simulink model "No"  (R2018b)
settings: Solver=VariableStepAuto  StartTime=0.0  StopTime=10.0  RelTol=1e-3
settings Model: Creator=kekos  LastModifiedBy=kekos

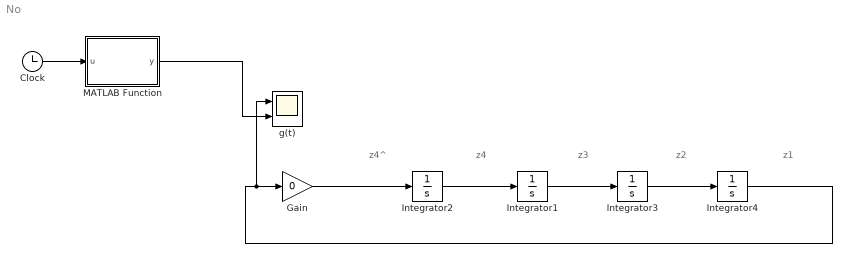
== system No ==
  note: z1
  note: z2
  note: z3
  note: z4
  note: z4^
  Clock : Clock
  Gain : Gain  Gain=0
  Integrator1 : Integrator
  Integrator2 : Integrator  InitialCondition=18
  Integrator3 : Integrator  InitialCondition=2
  Integrator4 : Integrator  InitialCondition=1
  MATLAB Function : MATLAB Function  TreatAsAtomicUnit=on
  g(t) : Scope  NumInputPorts=2
  wires:
  MATLAB Function/1(y) -> g(t)/2
  Clock/1 -> MATLAB Function/1(u)
  Gain/1 -> Integrator2/1
  Integrator2/1 -> Integrator1/1
  Integrator1/1 -> Integrator3/1
  Integrator3/1 -> Integrator4/1
  Integrator4/1 -> g(t)/1, Gain/1

== matlab function No/MATLAB Function ==
  data: u input; y output
function y = fcn(u)

y = 1+2*u+3*u^3;
